simulink model "mdlref_counter_bus_qnx"  (R2013a)
settings: Solver=FixedStepDiscrete  StartTime=0.0  StopTime=30.0  FixedStep=0.1  RelTol=1e-3
PreLoadFcn:
  | load sldemo_mdlref_counter_bus.mat
settings Model: SimulationMode=external  ExtModeAutoUpdateStatusClock=off  Creator=The MathWorks Inc.  LastModifiedBy=peselnikmg
settings DataIOCC: ExternalInput=topOut.getElement('COUNTERBUS'), topOut.getElement('INCREMENTBUS')  LoadExternalInput=on  SaveFormat=StructureWithTime  SaveOutput=off  SaveTime=off  SignalLoggingName=subOut
settings OptimizationCC: InlineParams=on  InlineInvariantSignals=on  ExpressionDepthLimit=2147483647  ZeroExternalMemoryAtStartup=off  ZeroInternalMemoryAtStartup=off  NoFixptDivByZeroProtection=on  EfficientFloat2IntCast=on  OptimizeModelRefInitCode=on  LifeSpan=1  BufferReusableBoundary=off
settings DebuggingCC: SaveWithParameterizedLinksMsg=none  CheckExecutionContextPreStartOutputMsg=on  CheckExecutionContextRuntimeOutputMsg=on  SolverPrmCheckMsg=none  MultiTaskDSMMsg=warning  MultiTaskCondExecSysMsg=none  SigSpecEnsureSampleTimeMsg=none  FcnCallInpInsideContextMsg=UseLocalSettings  BusObjectLabelMismatch=error  ModelReferenceDataLoggingMessage=none  StrictBusMsg=ErrorOnBusTreatedAsVector
settings HardwareCC: TargetHWDeviceType=32-bit Generic
settings ModelReferenceCC: UpdateModelReferenceTargets=IfOutOfDate  CheckModelReferenceTargetMessage=none
settings RTWCC: SystemTargetFile=ert_qnx.tlc  TemplateMakefile=ert_qnx.tmf  PostCodeGenCommand=postGenFunc(buildInfo)  Description=Embedded Coder  GenerateReport=on  ProcessScript=ert_qnx_make_rtw_hook  IncludeHyperlinkInReport=on  LaunchReport=on  IncludeERTFirstTime=on
settings CodeAppCC: IgnoreCustomStorageClasses=off  MaxIdLength=100
settings STFCustomTargetCC: TargetLibSuffix=.a  GenerateSampleERTMain=on  CompOptLevelCompliant=on  IncludeMdlTerminateFcn=off  CombineOutputUpdateFcns=on  ERTFirstTimeCompliant=on  ERTCustomFileBanners=on  SupportNonFinite=off  SupportContinuousTime=off  SupportNonInlinedSFcns=off  MATLABClassNameForMDSCustomization=Simulink.SoftwareTarget.ERTCustomization  SystemTargetFile=ert_qnx.tlc
settings ERTTargetCC: ParMdlRefBuildCompliant=off  ConcurrentExecutionCompliant=off  IncludeMdlTerminateFcn=off  SupportNonFinite=off  ModelStepFunctionPrototypeControlCompliant=off  CPPClassGenCompliant=off  ExtMode=on  ExtModeMexArgs=getpref('qnx_ert','TargetIP') 1 17725  TargetOS=VxWorksExample  ERTCustomFileTemplate=qnx_file_process.tlc

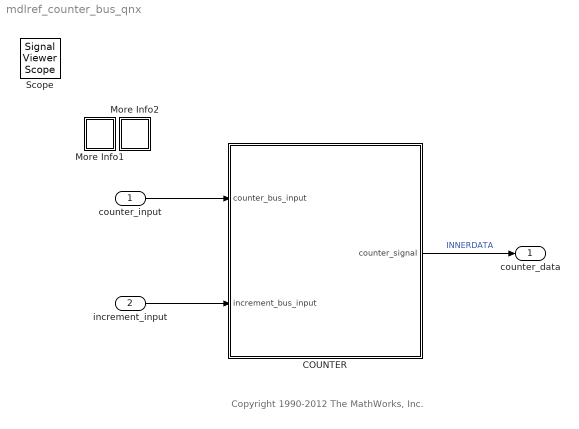
== system mdlref_counter_bus_qnx ==
  note: Copyright 1990-2012 The MathWorks, Inc.
  counter_input : Inport  OutDataTypeStr=Bus: COUNTERBUS  PortDimensions=[2 1]  BusOutputAsStruct=on
  increment_input : Inport  Port=2  OutDataTypeStr=Bus: INCREMENTBUS  PortDimensions=1  BusOutputAsStruct=on
  COUNTER : Subsystem
  More Info1 : Subsystem
      settings: OpenFcn=showdemo('sldemo_mdlref_bus')
      mask Display: disp('?')
  More Info2 : Subsystem
      settings: OpenFcn=|
      | html = fullfile(matlabroot, 'toolbox', 'simulink', 'simdemos', 'simfeatures', 'html', 'sldemo_mdlref_protect.html');
      | 
      | if(isempty(dir(html)))
      |    error('simdemos:sldemo_mdlref_bus:notFound','"%s" not found.',html);
      | else
      |    web(html, '-helpbrowser');
      | end
      mask Display: disp('?')
  counter_data : Outport
  Scope : SignalViewerScope  IOType=viewer  RefreshTime=0.035000
      settings: ShowLegends=on  YMax=45
  wires:
  counter_input/1 -> COUNTER/1(counter_bus_input)
  increment_input/1 -> COUNTER/2(increment_bus_input)
  COUNTER/1(counter_signal) -> counter_data/1  "INNERDATA"

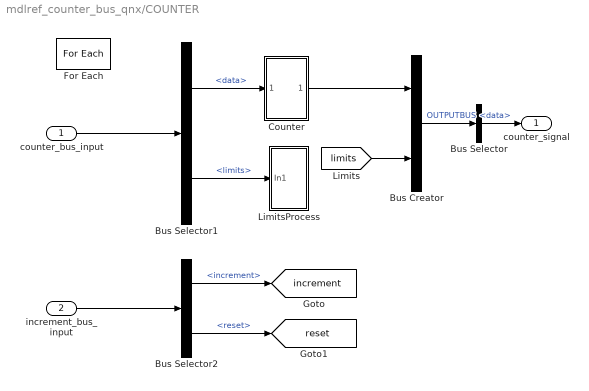
== system mdlref_counter_bus_qnx/COUNTER ==
  counter_bus_input : Inport  OutDataTypeStr=Bus: COUNTERBUS  Partition=on  PartitionDimension=1  PartitionWidth=1
  increment_bus_input : Inport  Port=2  OutDataTypeStr=Bus: INCREMENTBUS  Partition=off
  Bus Creator : BusCreator  Inputs=2  OutDataTypeStr=Bus: COUNTERBUS  NonVirtualBus=on
  Bus Selector : BusSelector  OutputSignals=data
  Bus Selector1 : BusSelector  OutputSignals=data,limits
  Bus Selector2 : BusSelector  OutputSignals=increment,reset
  Counter : Subsystem
  For Each : ForEach  DisableCoverage=on  IndexMode=One-based
  LimitsProcess : Subsystem
  counter_signal : Outport  ConcatenationDimension=1
  tag scope: increment=global, reset=global
  wires:
  Bus Creator/1 -> Bus Selector/1  "OUTPUTBUS"
  Counter/1(Out1) -> Bus Creator/1
  increment_bus_input/1 -> Bus Selector2/1
  Bus Selector1/2 -> LimitsProcess/1(In1)  "<limits>"
  Bus Selector1/1 -> Counter/1(In1)  "<data>"
  [limits] -> Bus Creator/2
  counter_bus_input/1 -> Bus Selector1/1
  Bus Selector2/2 -> [reset]  "<reset>"
  Bus Selector2/1 -> [increment]  "<increment>"
  Bus Selector/1 -> counter_signal/1  "<data>"

== system mdlref_counter_bus_qnx/More Info1 ==
  note: This demonstration shows how signals may be grouped and ungrouped while
      | retaining their names.  In this demonstration, 5 signals are created and labeled
      | appropriately.  These signals are then grouped together to create a bus of signals.
      | This bus of signals is then fed into the Bus Selector block.  Inside of the Bus
      | Selector block, the Pulse and Chirp signals are chosen to be output from the
      | original signal bus.
      |
      | It is possible to place a nest signal buses and then still retrieve the original signal
      | with its label.
  note: Bus Block Demonstration

== system mdlref_counter_bus_qnx/More Info2 ==
  note: Bus Block Demonstration
  note: This demonstration shows how signals may be grouped and ungrouped while
      | retaining their names.  In this demonstration, 5 signals are created and labeled
      | appropriately.  These signals are then grouped together to create a bus of signals.
      | This bus of signals is then fed into the Bus Selector block.  Inside of the Bus
      | Selector block, the Pulse and Chirp signals are chosen to be output from the
      | original signal bus.
      |
      | It is possible to place a nest signal buses and then still retrieve the original signal
      | with its label.

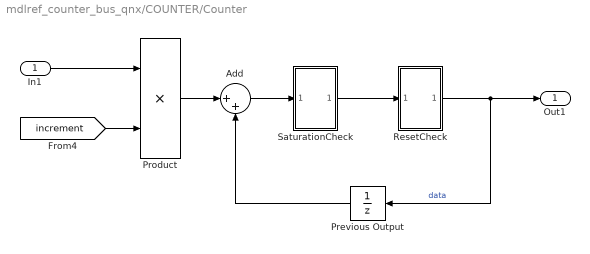
== system mdlref_counter_bus_qnx/COUNTER/Counter ==
  In1 : Inport
  Add : Sum  Inputs=|++
  Previous Output : UnitDelay  SampleTime=-1
  Product : Product  OutDataTypeStr=int32  RndMeth=Zero
  ResetCheck : Subsystem
  SaturationCheck : Subsystem
  Out1 : Outport
  wires:
  SaturationCheck/1(Out1) -> ResetCheck/1(In1)
  Previous Output/1 -> Add/2
  Add/1 -> SaturationCheck/1(In1)
  ResetCheck/1(Out2) -> Out1/1, Previous Output/1  "data"
  In1/1 -> Product/1
  [increment] -> Product/2
  Product/1 -> Add/1

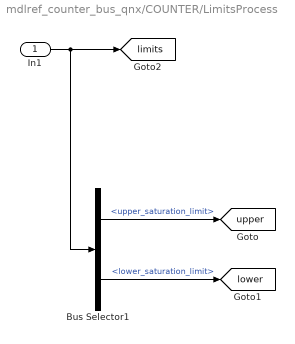
== system mdlref_counter_bus_qnx/COUNTER/LimitsProcess ==
  In1 : Inport
  Bus Selector1 : BusSelector  OutputSignals=upper_saturation_limit,lower_saturation_limit
  tag scope: limits=global, lower=global, upper=global
  wires:
  In1/1 -> Bus Selector1/1, [limits]
  Bus Selector1/2 -> [lower]  "<lower_saturation_limit>"
  Bus Selector1/1 -> [upper]  "<upper_saturation_limit>"

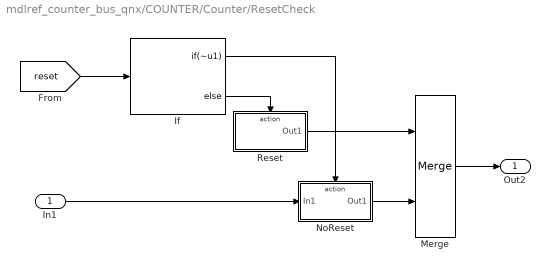
== system mdlref_counter_bus_qnx/COUNTER/Counter/ResetCheck ==
  In1 : Inport
  If : If  IfExpression=~u1
  Merge : Merge
  NoReset : Subsystem  TreatAsAtomicUnit=on
  Reset : Subsystem  TreatAsAtomicUnit=on
  Out2 : Outport
  wires:
  [reset] -> If/1
  If/1 -> NoReset/Action
  In1/1 -> NoReset/1(In1)
  If/2 -> Reset/Action
  Merge/1 -> Out2/1
  Reset/1(Out1) -> Merge/1
  NoReset/1(Out1) -> Merge/2

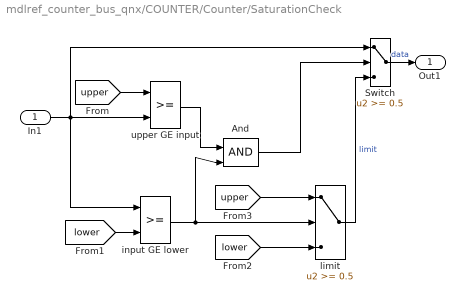
== system mdlref_counter_bus_qnx/COUNTER/Counter/SaturationCheck ==
  In1 : Inport
  " input GE lower" : RelationalOperator  Priority=1  OutDataTypeStr=boolean  InputSameDT=on
      settings: AttributesFormatString=\n
  And : Logic  IconShape=distinctive  OutDataTypeStr=boolean
  Switch : Switch  Threshold=0.5  SaturateOnIntegerOverflow=on  InputSameDT=on
  limit : Switch  Threshold=0.5  SaturateOnIntegerOverflow=on  InputSameDT=on
  upper GE input : RelationalOperator  Priority=0  OutDataTypeStr=boolean  InputSameDT=on
      settings: AttributesFormatString=\n
  Out1 : Outport
  wires:
  [upper] -> limit/1
  limit/1 -> Switch/3  "limit"
  upper GE input/1 -> And/1
  [lower] -> limit/3
  [upper] -> upper GE input/1
  [lower] -> " input GE lower"/2
  " input GE lower"/1 -> And/2, limit/2
  And/1 -> Switch/2
  In1/1 -> Switch/1, upper GE input/2, " input GE lower"/1
  Switch/1 -> Out1/1  "data"

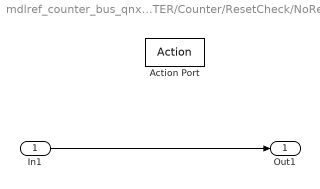
== system mdlref_counter_bus_qnx/COUNTER/Counter/ResetCheck/NoReset ==
  In1 : Inport
  Action Port : ActionPort  ActionType=then
  Out1 : Outport
  wires:
  In1/1 -> Out1/1

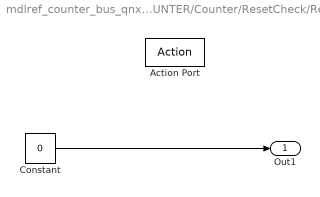
== system mdlref_counter_bus_qnx/COUNTER/Counter/ResetCheck/Reset ==
  Action Port : ActionPort  ActionType=else
  Constant : Constant  Value=0  OutDataTypeStr=int32
  Out1 : Outport  InitialOutput=0
  wires:
  Constant/1 -> Out1/1
